simulink model "wiper_prpject_second_way"  (R2021a)
settings: Solver=FixedStepAuto  StartTime=0.0  StopTime=20  FixedStep=0.01  RelTol=1e-3
model workspace (MAT data in the model file):
  Sig = Simulink.Signal
  Sig.DataType = 'auto'
  Sig.Dimensions = -1
  Sig.DimensionsMode = 'auto'
  Sig.Complexity = 'auto'
  Sig.SampleTime = -1
  Sig.SamplingMode = 'auto'
  x_data_table = Simulink.Parameter
  x_data_table.Value = [0 1 2 3 4 5 6 7]
  x_data_table.DataType = 'auto'
  x_data_table.Dimensions = [1 8]
  y_data_table = Simulink.Parameter
  y_data_table.Value = [0 0.4 0.45 0.5 0.55 0.6 0.65 0.75]
  y_data_table.DataType = 'auto'
  y_data_table.Dimensions = [1 8]
undefined symbols (not defined in the file): sigbuilder_block
libraries: simulink x2
settings Model: Creator=Beshary  LastModifiedBy=Beshary
settings OptimizationCC: DefaultUnderspecifiedDataType=single

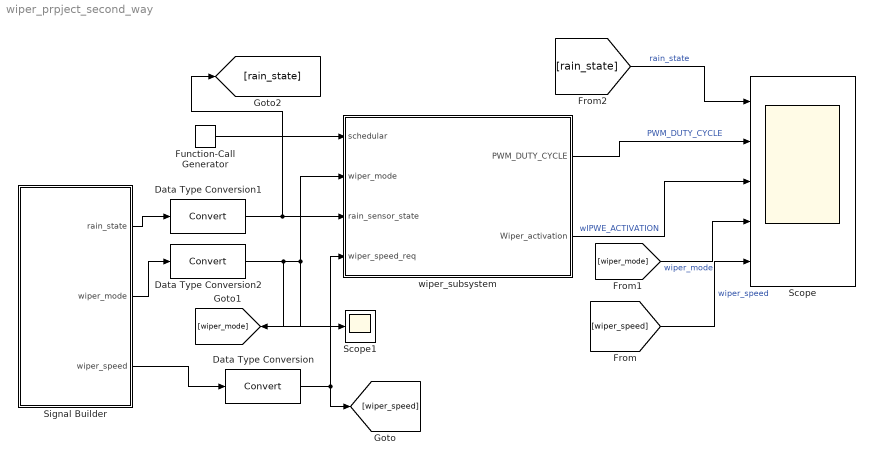
== system wiper_prpject_second_way ==
  Data Type Conversion : DataTypeConversion
  Data Type Conversion1 : DataTypeConversion
  Data Type Conversion2 : DataTypeConversion
  Function-Call Generator : simulink/Ports & Subsystems/Function-Call Generator  sample_time=0.01  numberOfIterations=1  DisallowWideOutput=off
  Scope : Scope  NumInputPorts=5
  Scope1 : Scope
  Signal Builder : Subsystem  Tag=STV Subsys  LoadFcn=sigbuilder_block('load');  StartFcn=sigbuilder_block('start');  StopFcn=sigbuilder_block('stop');  ClipboardFcn=sigbuilder_block('clipboard');  mask(Sigbuilder block){tuvar=[0:10]}
      mask help: Simulink:masks:SigbuilderBlock_MD
      mask init:
      | if ~strcmp(get_param(bdroot(gcbh),'SimulationStatus'),'stopped') tuvar = sigbuilder_block('maskInit'); end
      settings: CopyFcn=sigbuilder_block('copy');  DeleteFcn=sigbuilder_block('delete');  ModelCloseFcn=sigbuilder_block('modelClose');  PreSaveFcn=sigbuilder_block('preSave');  PauseFcn=sigbuilder_block('pause');  ContinueFcn=sigbuilder_block('continue');  NameChangeFcn=sigbuilder_block('namechange');  OpenFcn=sigbuilder_block('open',[5.4 30 1141.2 522.6 ]);  CloseFcn=sigbuilder_block('close');
      mask Display: plot(0, 0, 100, 100,[2, 2, 32, 32, 2], [68, 8, 8, 68, 68],[32, 2], [38, 38], [32, 19, 2],[53, 60, 44], [32, 17, 17, 2],[16, 16, 31, 31]);txt = getActiveGroup(gcbh);text(2, 100, txt,'verticalAlignment', 'top');
  wiper_subsystem : Subsystem
  wires:
  Signal Builder/2(wiper_mode) -> Data Type Conversion2/1
  Data Type Conversion2/1 -> Scope1/1, [wiper_mode], wiper_subsystem/2(wiper_mode)
  [rain_state] -> Scope/1  "rain_state"
  Signal Builder/1(rain_state) -> Data Type Conversion1/1
  Data Type Conversion/1 -> wiper_subsystem/4(wiper_speed_req), [wiper_speed]
  wiper_subsystem/1(PWM_DUTY_CYCLE) -> Scope/2  "PWM_DUTY_CYCLE"
  wiper_subsystem/2(Wiper_activation) -> Scope/3  "wIPWE_ACTIVATION"
  Function-Call Generator/1 -> wiper_subsystem/1(schedular)
  Signal Builder/3(wiper_speed) -> Data Type Conversion/1
  [wiper_mode] -> Scope/4  "wiper_mode"
  [wiper_speed] -> Scope/5  "wiper_speed"
  Data Type Conversion1/1 -> [rain_state], wiper_subsystem/3(rain_sensor_state)

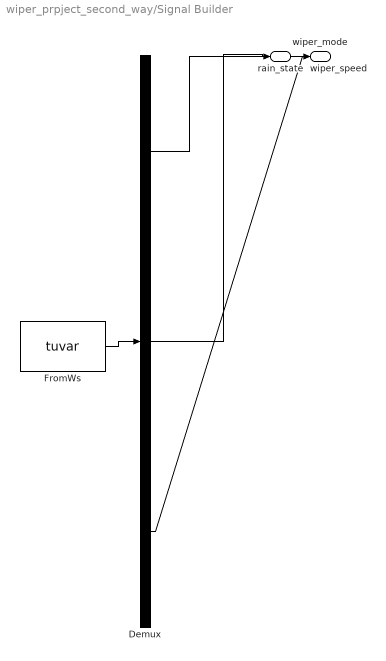
== system wiper_prpject_second_way/Signal Builder ==
  Demux : Demux  Tag=STV Demux  Outputs=3
      settings: DisplayOption=none
  FromWs : FromWorkspace  Tag=STV FromWs  VariableName=tuvar
      SigBuilderData=|
      | common.afterFinalStr = 'Extrapolate'
      | common.sampleTime = 0
      | dataSet.timeRange = [0 20]
      | dataSet.name = 'Group 1'
      | sbobj.Groups.Name = 'Group 1'
      | sbobj.Groups.Signals(1).Name = 'rain_state'
      | sbobj.Groups.Signals(1).XData = [0 4 6 14 15 16 20]
      | sbobj.Groups.Signals(1).YData = [0 0 0 0 1 0 0]
      | sbobj.Groups.Signals(2).Name = 'wiper_mode'
      | sbobj.Groups.Signals(2).XData = [0 0.96 2 3 4 5 6 20]
      | sbobj.Groups.Signals(2).YData = [0 0 2 2 3 3 1 1]
      | sbobj.Groups.Signals(3).Name = 'wiper_speed'
      | sbobj.Groups.Signals(3).XData = [0 7 13.98 20]
      | sbobj.Groups.Signals(3).YData = [0 0 7 7]
      | sbobj.Groups.TimeRange = [0 20]
  rain_state : Outport  Tag=STV Outport
  wiper_mode : Outport  Tag=STV Outport  Port=2
  wiper_speed : Outport  Tag=STV Outport  Port=3
  wires:
  Demux/1 -> rain_state/1
  FromWs/1 -> Demux/1
  Demux/2 -> wiper_mode/1
  Demux/3 -> wiper_speed/1

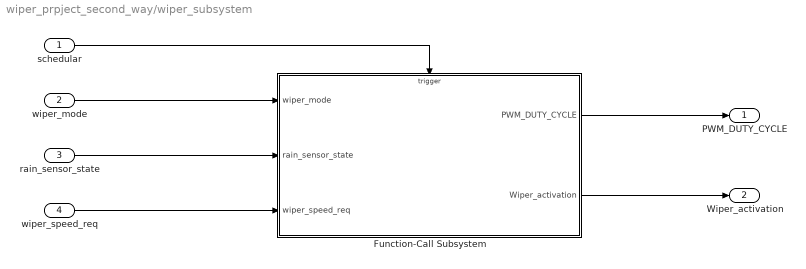
== system wiper_prpject_second_way/wiper_subsystem ==
  schedular : Inport
  wiper_mode : Inport  Port=2  OutDataTypeStr=uint16
  rain_sensor_state : Inport  Port=3  OutDataTypeStr=boolean
  wiper_speed_req : Inport  Port=4  OutDataTypeStr=uint8
  Function-Call Subsystem : Subsystem  TreatAsAtomicUnit=on
  PWM_DUTY_CYCLE : Outport  OutDataTypeStr=single
  Wiper_activation : Outport  Port=2  OutDataTypeStr=boolean
  wires:
  schedular/1 -> Function-Call Subsystem/Trigger
  wiper_mode/1 -> Function-Call Subsystem/1(wiper_mode)
  rain_sensor_state/1 -> Function-Call Subsystem/2(rain_sensor_state)
  wiper_speed_req/1 -> Function-Call Subsystem/3(wiper_speed_req)
  Function-Call Subsystem/1(PWM_DUTY_CYCLE) -> PWM_DUTY_CYCLE/1
  Function-Call Subsystem/2(Wiper_activation) -> Wiper_activation/1

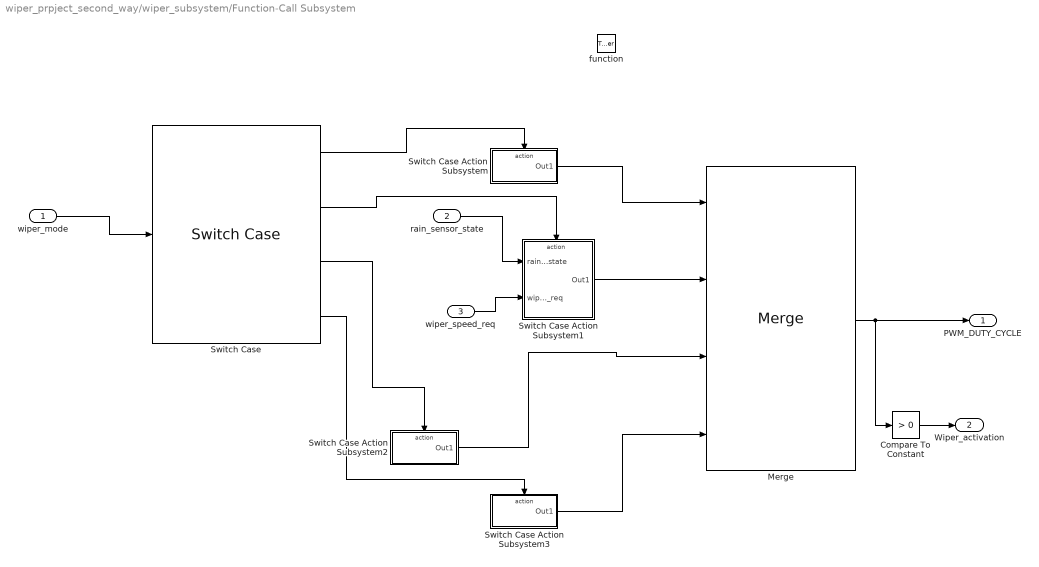
== system wiper_prpject_second_way/wiper_subsystem/Function-Call Subsystem ==
  wiper_mode : Inport  OutDataTypeStr=uint16
  rain_sensor_state : Inport  Port=2  OutDataTypeStr=boolean
  wiper_speed_req : Inport  Port=3
  function : TriggerPort  TriggerType=function-call  VariantControl=(inherit)
  Compare To Constant : simulink/Logic and Bit Operations/Compare To Constant  relop=>  const=0  OutDataTypeStr=boolean
  Merge : Merge  Inputs=4
  Switch Case : SwitchCase  CaseConditions={0,1,2,3}  ShowDefaultCase=off
  Switch Case Action Subsystem : Subsystem  TreatAsAtomicUnit=on
  Switch Case Action Subsystem1 : Subsystem  TreatAsAtomicUnit=on
  Switch Case Action Subsystem2 : Subsystem  TreatAsAtomicUnit=on
  Switch Case Action Subsystem3 : Subsystem  TreatAsAtomicUnit=on
  PWM_DUTY_CYCLE : Outport
  Wiper_activation : Outport  Port=2
  wires:
  Switch Case/1 -> Switch Case Action Subsystem/Action
  Switch Case/2 -> Switch Case Action Subsystem1/Action
  Switch Case/3 -> Switch Case Action Subsystem2/Action
  Switch Case/4 -> Switch Case Action Subsystem3/Action
  wiper_mode/1 -> Switch Case/1
  Switch Case Action Subsystem/1(Out1) -> Merge/1
  Switch Case Action Subsystem1/1(Out1) -> Merge/2
  Switch Case Action Subsystem2/1(Out1) -> Merge/3
  Switch Case Action Subsystem3/1(Out1) -> Merge/4
  Merge/1 -> Compare To Constant/1, PWM_DUTY_CYCLE/1
  rain_sensor_state/1 -> Switch Case Action Subsystem1/1(rain_sensor_state)
  wiper_speed_req/1 -> Switch Case Action Subsystem1/2(wiper_speed_req)
  Compare To Constant/1 -> Wiper_activation/1

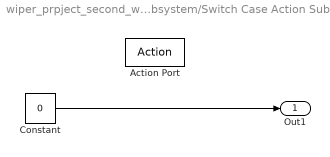
== system wiper_prpject_second_way/wiper_subsystem/Function-Call Subsystem/Switch Case Action Subsystem ==
  Action Port : ActionPort  ActionPortLabel=case [ 0 ]:
  Constant : Constant  Value=0  OutDataTypeStr=single
  Out1 : Outport  OutDataTypeStr=single
  wires:
  Constant/1 -> Out1/1

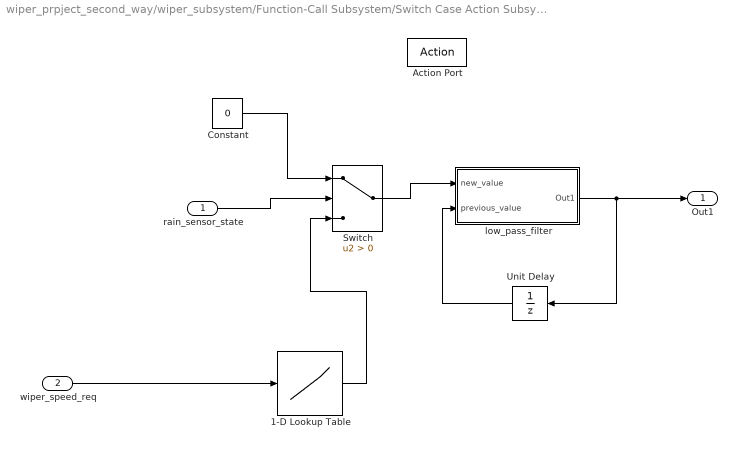
== system wiper_prpject_second_way/wiper_subsystem/Function-Call Subsystem/Switch Case Action Subsystem1 ==
  rain_sensor_state : Inport  OutDataTypeStr=boolean
  wiper_speed_req : Inport  Port=2
  Action Port : ActionPort  ActionPortLabel=case [ 1 ]:
  1-D Lookup Table : Lookup_n-D  NumberOfTableDimensions=1  BreakpointsForDimension1=x_data_table  Table=y_data_table  TableDataTypeStr=single  InterpMethod=Nearest  InternalRulePriority=Speed  OutDataTypeStr=single  RndMeth=Simplest  InputSameDT=on
  Constant : Constant  Value=0  OutDataTypeStr=single
  Switch : Switch  Criteria=u2 > Threshold
  Unit Delay : UnitDelay  SampleTime=-1  HasFrameUpgradeWarning=on
  low_pass_filter : Subsystem
  Out1 : Outport  OutDataTypeStr=single
  wires:
  rain_sensor_state/1 -> Switch/2
  Constant/1 -> Switch/1
  Switch/1 -> low_pass_filter/1(new_value)
  wiper_speed_req/1 -> 1-D Lookup Table/1
  low_pass_filter/1(Out1) -> Unit Delay/1, Out1/1
  1-D Lookup Table/1 -> Switch/3
  Unit Delay/1 -> low_pass_filter/2(previous_value)

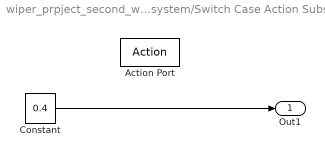
== system wiper_prpject_second_way/wiper_subsystem/Function-Call Subsystem/Switch Case Action Subsystem2 ==
  Action Port : ActionPort  ActionPortLabel=case [ 2 ]:
  Constant : Constant  Value=0.4  OutDataTypeStr=single
  Out1 : Outport  OutDataTypeStr=single
  wires:
  Constant/1 -> Out1/1

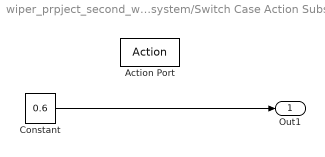
== system wiper_prpject_second_way/wiper_subsystem/Function-Call Subsystem/Switch Case Action Subsystem3 ==
  Action Port : ActionPort  ActionPortLabel=case [ 3 ]:
  Constant : Constant  Value=0.6  OutDataTypeStr=single
  Out1 : Outport  OutDataTypeStr=single
  wires:
  Constant/1 -> Out1/1

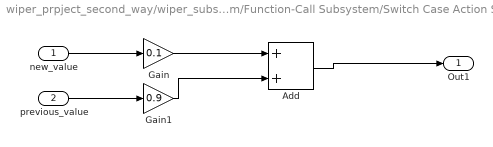
== system wiper_prpject_second_way/wiper_subsystem/Function-Call Subsystem/Switch Case Action Subsystem1/low_pass_filter ==
  new_value : Inport  OutDataTypeStr=single
  previous_value : Inport  Port=2
  Add : Sum  AccumDataTypeStr=single  OutDataTypeStr=single
  Gain : Gain  Gain=0.1  ParamDataTypeStr=single  OutDataTypeStr=single
  Gain1 : Gain  Gain=0.9
  Out1 : Outport  OutDataTypeStr=single
  wires:
  new_value/1 -> Gain/1
  previous_value/1 -> Gain1/1
  Gain1/1 -> Add/2
  Gain/1 -> Add/1
  Add/1 -> Out1/1
